simulink model "maneuver_generator"  (R2016b)
settings: Solver=FixedStepAuto  StartTime=0.0  StopTime=9  FixedStep=1  RelTol=1e-3
values from neighbouring files (symbols this model uses):
  fk = fk+r    [run.m]
libraries: aerolibptmass x1
settings Model: Creator=hyPar  LastModifiedBy=hyPar

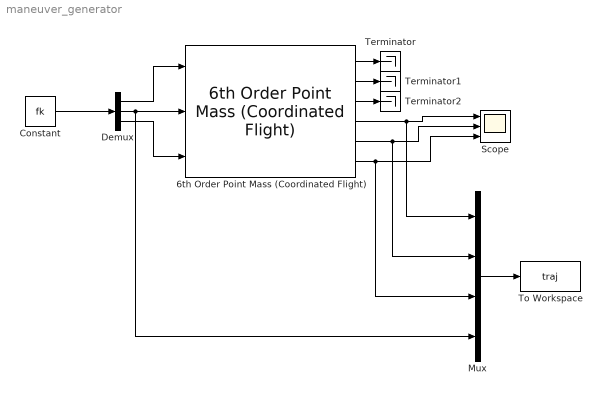
== system maneuver_generator ==
  6th Order Point Mass (Coordinated Flight) : aerolibptmass/6th Order Point Mass (Coordinated Flight)  units=Metric (MKS)  gamma0=0  chi0=0  V0=200  x0=0  y0=0  h0=5000  mass0=1000.0
  Constant : Constant  Value=fk
  Demux : Demux  Outputs=3
  Mux : Mux
  Scope : Scope  NumInputPorts=3
  Terminator : Terminator
  Terminator1 : Terminator
  Terminator2 : Terminator
  To Workspace : ToWorkspace  VariableName=traj  SaveFormat=Timeseries  SampleTime=-1
  wires:
  6th Order Point Mass (Coordinated Flight)/4 -> Scope/1, Mux/1
  6th Order Point Mass (Coordinated Flight)/5 -> Mux/2, Scope/2
  6th Order Point Mass (Coordinated Flight)/6 -> Mux/3, Scope/3
  Constant/1 -> Demux/1
  Demux/1 -> 6th Order Point Mass (Coordinated Flight)/1
  Demux/2 -> Mux/4, 6th Order Point Mass (Coordinated Flight)/2
  Demux/3 -> 6th Order Point Mass (Coordinated Flight)/3
  Mux/1 -> To Workspace/1
  6th Order Point Mass (Coordinated Flight)/2 -> Terminator1/1
  6th Order Point Mass (Coordinated Flight)/3 -> Terminator2/1
  6th Order Point Mass (Coordinated Flight)/1 -> Terminator/1
